simulink model "J3"  (R2019b)
settings: Solver=VariableStepAuto  StartTime=0.0  StopTime=10.0  RelTol=1e-3
settings Model: Creator=Inspiron  LastModifiedBy=Inspiron

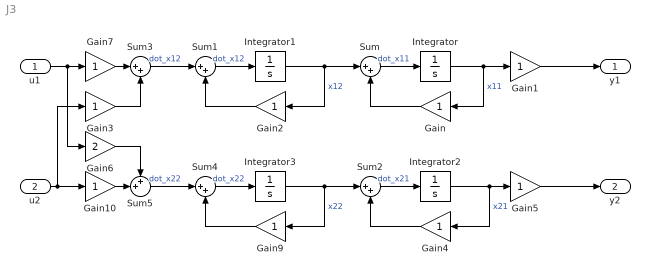
== system J3 ==
  u1 : Inport
  u2 : Inport  Port=2
  Gain{,1..5,7,9..10} (9 alike) : Gain
  Gain6 : Gain  Gain=2
  Integrator{,1..3} (4 alike) : Integrator
  Sum{,1..4} (5 alike) : Sum  Inputs=|++
  Sum5 : Sum  Inputs=++|
  y1 : Outport
  y2 : Outport  Port=2
  wires:
  u1/1 -> Gain6/1, Gain7/1
  Gain5/1 -> y2/1
  Gain1/1 -> y1/1
  Integrator2/1 -> Gain4/1, Gain5/1  "x21"
  Sum2/1 -> Integrator2/1  "dot_x21"
  Sum1/1 -> Integrator1/1  "dot_x12"
  Integrator1/1 -> Sum/1, Gain2/1  "x12"
  Integrator/1 -> Gain1/1, Gain/1  "x11"
  Sum/1 -> Integrator/1  "dot_x11"
  Gain/1 -> Sum/2
  Gain2/1 -> Sum1/2
  Sum4/1 -> Integrator3/1  "dot_x22"
  Integrator3/1 -> Sum2/1, Gain9/1  "x22"
  Gain9/1 -> Sum4/2
  Gain4/1 -> Sum2/2
  u2/1 -> Gain3/1, Gain10/1
  Gain7/1 -> Sum3/1
  Sum3/1 -> Sum1/1  "dot_x12"
  Sum5/1 -> Sum4/1  "dot_x22"
  Gain10/1 -> Sum5/2
  Gain6/1 -> Sum5/1
  Gain3/1 -> Sum3/2
